simulink library "MPCMdlLib"  (Simulink 7.1)
undefined symbols (not defined in the file or in its folder): CombineFandG, GetBlockName, getfullname, sparse, x1, x2
libraries: MPCMdlLib x8
settings Model: Creator=Serg  LastModifiedBy=serg

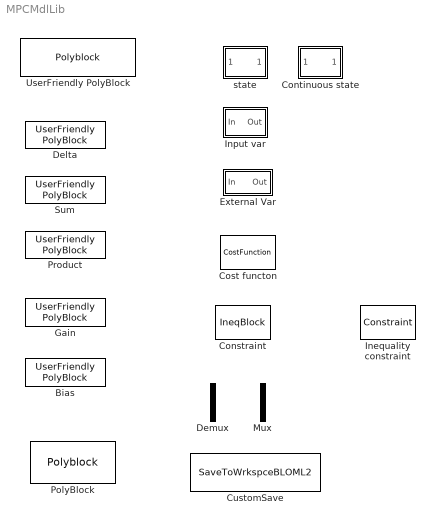
== system MPCMdlLib ==
  Bias : MPCMdlLib/UserFriendly PolyBlock  Tag=PolyBlock  A="[1   ; 0  ]"  C="[1  2]"  gA=[ 0]  gC=1  input_type=Scalar  output_type=Scalar  port_names=u
  Constraint : M-S-Function  Tag=InequalBlock  FunctionName=IneqBlock  Parameters=CompareSign  mask{CompareSign=< 0}
      mask prompts: CompareSign "Sign"
      mask init:
      | if (CompareSign == 1)
      |     strtitle = '< 0 ';
      | else
      |     strtitle = '> 0 ';
      | end
      mask StyleString: popup(< 0|> 0)
      mask Display: fprintf(strtitle);
  Continuous state : Subsystem  Tag=OptState  InitFcn=set_param(getfullname(gcb),'save_name', GetBlockName(gcb))  mask{init_val=0, save_name=vvmodel_state1}
      mask prompts: init_val "Initial value"
      mask Display: fprintf('1/s')
  Cost functon : M-S-Function  Tag=OptCost  FunctionName=CostFunction
      mask Display:
      | port_label('input',1,'in');
      | 
      | 
      | text(0.5,0.5,'\Sigma','texmode','on');
  CustomSave : M-S-Function  FunctionName=SaveToWrkspceBLOML2  Parameters='name'
  Delta : MPCMdlLib/UserFriendly PolyBlock  Tag=PolyBlock  A="[1  0  ; 0 1 ]"  C="[1  -1]"  gA=[0 0]  gC=1  input_type=Scalar  output_type=Scalar  port_names=x1,x2
  Demux : Demux  Outputs=2
  External Var : Subsystem  Tag=OptExternal  InitFcn=set_param(getfullname(gcb),'save_name', GetBlockName(gcb))  mask{save_name=0}
      mask prompts: save_name "Name to save"
      mask Display: fprintf('External')
  Gain : MPCMdlLib/UserFriendly PolyBlock  Tag=PolyBlock  A="[1   ]"  C=[2 ]  gA=[0 ]  gC=1  input_type=Scalar  output_type=Scalar  port_names=u
  Inequality constraint : MPCMdlLib/Constraint  Tag=InequalBlock  CompareSign=< 0
  Input var : Subsystem  Tag=OptInput  InitFcn=set_param(getfullname(gcb),'save_name', GetBlockName(gcb))  mask{step_ratio=1, save_name=0}
      mask prompts: step_ratio "Step ratio"; save_name "Name to save"
      mask Display: fprintf('Input')
  Mux : Mux  Inputs=2
  PolyBlock : M-S-Function  Tag=PolyBlock  FunctionName=Polyblock  Parameters=A, C , input_type, output_type  mask{A=sparse([1 0 ; 0  1]), C=sparse([1 -1]), input_type=Scalar, output_type=Scalar}
      mask prompts: A "A matrix"; C "C matrix"; input_type "Input as"; output_type "Output as"
      mask help:
      | Function of the form p(x,y)=0.
      | y is assumed to be m last variables, where m is size(C,1).
      mask StyleString: edit,edit,popup(Scalar|Vector),popup(Scalar|Vector)
  Product : MPCMdlLib/UserFriendly PolyBlock  Tag=PolyBlock  A="[1  1  ]"  C=[1 ]  gA=[0 0]  gC=1  input_type=Scalar  output_type=Scalar  port_names=x1,x2
  Sum : MPCMdlLib/UserFriendly PolyBlock  Tag=PolyBlock  A="[1  0  ; 0 1 ]"  C="[1  1]"  gA=[0 0]  gC=1  input_type=Scalar  output_type=Scalar  port_names=x1,x2
  UserFriendly PolyBlock : M-S-Function  Tag=PolyBlock  FunctionName=Polyblock  Parameters=CombineFandG(A,C,gA, gC,'A'),CombineFandG(A,C,gA, gC,'C'), input_type, output_type  mask{A=sparse([1  1 ]), C=sparse([1 ]), gA=[0 0 ], gC=1, input_type=Scalar, output_type=Scalar, port_names=x1,x2}
      mask prompts: A "A matrix for f"; C "C matrix for f"; gA "A matrix for g"; gC "C matrix for g"; input_type "Input as"; output_type "Output as"; port_names "Input names, comma separated"
      mask help:
      | y=f(x)/g(x)
      | Where f and g are sum of polinomial and exponential terms, described by A and C matrices.
      | Example: f=x1*exp(x3)+0.8*x1^3*x2
      | A = [1  0  inf ;
      |         3  1  0];
      | C = [1   0.8];
      mask init:
      | CheckACSizes(A,C,gA,gC)
      | 
      | pos = get_param(gcb,'position');
      | width = pos(3)-pos(1);
      | height = pos(4)-pos(2);
      | letter_width = 5; % pixels
      | letter_height = 15; % pixels
      | max_length = (width-15)/letter_width;
      | max_rows = max(1,floor((height-10)/letter_height));
      | 
      | remain = port_names;
      | i=0;
      | port_names_str = {};
      | while true
      |    [str, remain] = strtok(remain,',');
      |    if isempty(str),  break;  end
      |    if i >= size(A,2)
      |        break
      |    end
      |    i = i+1;
      |    port_names_str{i} = str;
      | %   disp(sprintf('%s', str))
      | end
      | %port_names_str
      | 
      | if (length(port_names_str) < size(A,2))
      |     for i= length(port_names_str)+1: size(A,2)
      |         port_names_str{i} = ['x' num2str(i)];
      |     end
      | end
      | 
      | 
      | 
      | names = port_names_str;
      | 
      | full_name = [];
      | for i = 1:min(size(C,1),max_rows)
      |     fname = CreatePolyFromMatrix(A,C(i,:),names,'low');
      |     if (length(fname) > max_length-5)
      |         fname = 'f(x)';
      |     end
      |     
      |     if (gC(1) == 1 && size(gA,1)==1 && sum(abs(gA(1,1:end)))==0)
      |         name = sprintf('%s',fname);
      |     else
      |         gname = CreatePolyFromMatrix(gA,gC,names,'low');
      |         name = sprintf('(%s)/(%s)',fname,gname);
      |         if (length(name) > max_length)
      |             
      |             gname = 'g(x)';
      |             name = sprintf('(%s)/%s',fname,gname);
      |         end
      |     end
      |     full_name = [full_name   name  char(10)];
      | end
      | 
      | 
      | labels = [ 'fprintf(full_name)' char(13) char(10) ];
      | if input_type == 1
      |     for idx = 1:length(port_names_str)
      |         thisLabel = sprintf('port_label(''input'',%d,''%s'')',idx,port_names_str{idx});
      |         labels = [labels thisLabel char(13) char(10)];
      |     end
      |     labels(end) = [];
      | end
      | set_param(gcb,'MaskDisplay',labels);
      settings: MoveFcn=set_param(gcb,'A',get_param(gcb,'A'))
      mask StyleString: edit,edit,edit,edit,popup(Scalar|Vector),popup(Scalar|Vector),edit
      mask Display:
      | fprintf(full_name)
      | port_label('input',1,'x1')
      | port_label('input',2,'x2')
  state : Subsystem  Tag=OptState  InitFcn=set_param(getfullname(gcb),'save_name', GetBlockName(gcb))  mask{init_val=0, save_name=vvmodel_state1}
      mask prompts: init_val "Initial value"
      mask Display: fprintf('1/z')

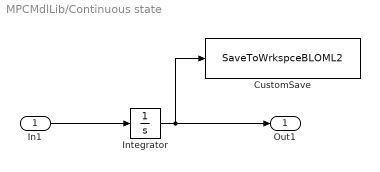
== system MPCMdlLib/Continuous state ==
  In1 : Inport  OutDataType=fixdt(1, 16)  OutScaling=2^0
  CustomSave : M-S-Function  FunctionName=SaveToWrkspceBLOML2  Parameters=name_to_save  mask{name_to_save=save_name}
      mask prompts: name_to_save "Variabke name"
  Integrator : Integrator  InitialCondition=init_val
  Out1 : Outport  OutDataType=fixdt(1, 16)  OutScaling=2^0
  wires:
  Integrator/1 -> CustomSave/1, Out1/1
  In1/1 -> Integrator/1

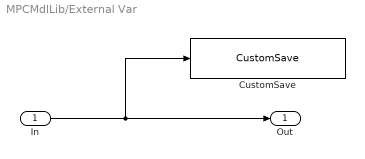
== system MPCMdlLib/External Var ==
  In : Inport  OutDataType=fixdt(1, 16)  OutScaling=2^0
  CustomSave : MPCMdlLib/state/CustomSave  name_to_save=save_name
  Out : Outport  OutDataType=fixdt(1, 16)  OutScaling=2^0
  wires:
  In/1 -> Out/1, CustomSave/1

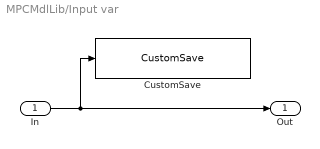
== system MPCMdlLib/Input var ==
  In : Inport  OutDataType=fixdt(1, 16)  OutScaling=2^0
  CustomSave : MPCMdlLib/state/CustomSave  name_to_save=save_name
  Out : Outport  OutDataType=fixdt(1, 16)  OutScaling=2^0
  wires:
  In/1 -> Out/1, CustomSave/1

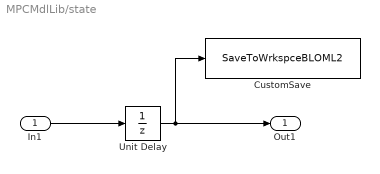
== system MPCMdlLib/state ==
  In1 : Inport  OutDataType=fixdt(1, 16)  OutScaling=2^0
  CustomSave : M-S-Function  FunctionName=SaveToWrkspceBLOML2  Parameters=name_to_save  mask{name_to_save=save_name}
      mask prompts: name_to_save "Variabke name"
  Unit Delay : UnitDelay  X0=init_val  SampleTime=-1
  Out1 : Outport  OutDataType=fixdt(1, 16)  OutScaling=2^0
  wires:
  In1/1 -> Unit Delay/1
  Unit Delay/1 -> Out1/1, CustomSave/1
